simulink model "P702_NI_SoftECU"  (R2019a)
settings: Solver=ode1  StartTime=0.0  StopTime=Inf  FixedStep=0.001  RelTol=1e-3  EnableMultiTasking=on
PreLoadFcn:
  | run '.\VeriStand_BlockSet\NIVeriStandAddPaths.m'
undefined symbols (not defined in the file or in its folder): magnitude
libraries: simulink x83, simulink_extras x1
(part 42 of 76)

== system P702_NI_SoftECU/Input/Carsim/Bus Conversion/MRR_BUS1 ==
  In1 : Inport
  Bus Creator : BusCreator  Inputs=12
  Bus Selector : BusSelector  OutputSignals=CAN_DET_RANGE_01[m],CAN_DET_RANGE_RATE_01[m/s],CAN_DET_AZIMUTH_01[rad],CAN_DET_ELEVATION_01[rad],CAN_DET_RANGE_02[m],CAN_DET_RANGE_RATE_02[m/s],CAN_DET_AZIMUTH_02[rad],CAN_DET_ELEVATION_02[rad],CAN_DET_RANGE_03[m],CAN_DET_RANGE_RATE_03[m/s],CAN_DET_AZIMUTH_03[rad],CAN_DET_ELEVATION_03[rad]
  Gain : Gain  Commented=through  Gain=1/3.6
  Gain10 : Gain  Commented=through  Gain=pi/180
  Gain11 : Gain
  Gain12 : Gain  Commented=through  Gain=1/3.6
  Gain13 : Gain
  Gain14 : Gain  Commented=through  Gain=1/3.6
  Gain3 : Gain
  Gain6 : Gain  Commented=through  Gain=pi/180
  Gain9 : Gain  Commented=through  Gain=pi/180
  Out1 : Outport
  wires:
  Bus Selector/1 -> Bus Creator/1  "<CAN_DET_RANGE_01[m]>"
  Bus Selector/11 -> Gain11/1  "<CAN_DET_AZIMUTH_03[rad]>"
  Bus Selector/3 -> Gain3/1  "<CAN_DET_AZIMUTH_01[rad]>"
  Bus Selector/2 -> Gain/1  "<CAN_DET_RANGE_RATE_01[m/s]>"
  Bus Selector/7 -> Gain13/1  "<CAN_DET_AZIMUTH_02[rad]>"
  Bus Selector/6 -> Gain14/1  "<CAN_DET_RANGE_RATE_02[m/s]>"
  Bus Selector/9 -> Bus Creator/9  "<CAN_DET_RANGE_03[m]>"
  Bus Selector/5 -> Bus Creator/5  "<CAN_DET_RANGE_02[m]>"
  Bus Creator/1 -> Out1/1
  In1/1 -> Bus Selector/1
  Bus Selector/4 -> Gain10/1  "<CAN_DET_ELEVATION_01[rad]>"
  Bus Selector/12 -> Gain6/1  "<CAN_DET_ELEVATION_03[rad]>"
  Bus Selector/8 -> Gain9/1  "<CAN_DET_ELEVATION_02[rad]>"
  Gain/1 -> Bus Creator/2  "CAN_DET_RANGE_RATE_01[m/s]"
  Gain3/1 -> Bus Creator/3  "CAN_DET_AZIMUTH_01[rad]"
  Gain10/1 -> Bus Creator/4  "CAN_DET_ELEVATION_01[rad]"
  Gain14/1 -> Bus Creator/6  "CAN_DET_RANGE_RATE_02[m/s]"
  Gain13/1 -> Bus Creator/7  "CAN_DET_AZIMUTH_02[rad]"
  Gain9/1 -> Bus Creator/8  "CAN_DET_ELEVATION_02[rad]"
  Gain12/1 -> Bus Creator/10  "CAN_DET_RANGE_RATE_03[m/s]"
  Gain11/1 -> Bus Creator/11  "CAN_DET_AZIMUTH_03[rad]"
  Gain6/1 -> Bus Creator/12  "CAN_DET_ELEVATION_03[rad]"
  Bus Selector/10 -> Gain12/1  "<CAN_DET_RANGE_RATE_03[m/s]>"

== system P702_NI_SoftECU/Input/Carsim/Bus Conversion/PCM_BUS ==
  In1 : Inport
  BrkLightSwtch_B : Constant  Value=0
  Bus Creator : BusCreator  Inputs=8
  Bus Selector : BusSelector  OutputSignals=Throttle[percentage],V_total_Vehicle[km/h],Engine_RPM[rpm],Gear[],T_Engine[Nm],a_x_veh_COG[g]
  CluBottomOfTravelSwtch_B : Constant  Value=0
  Gain : Gain  Gain=100
  Gain1 : Gain  Gain=9.8
  Out1 : Outport
  wires:
  In1/1 -> Bus Selector/1
  Gain/1 -> Bus Creator/1  "Throttle[percentage]"
  BrkLightSwtch_B/1 -> Bus Creator/8  "BrkLightSwtch_B"
  CluBottomOfTravelSwtch_B/1 -> Bus Creator/7  "CluBottomOfTravelSwtch_B"
  Bus Creator/1 -> Out1/1
  Bus Selector/5 -> Bus Creator/5  "<T_Engine[Nm]>"
  Bus Selector/4 -> Bus Creator/4  "<Gear[]>"
  Bus Selector/3 -> Bus Creator/3  "<Engine_RPM[rpm]>"
  Bus Selector/2 -> Bus Creator/2  "<V_total_Vehicle[km/h]>"
  Bus Selector/1 -> Gain/1  "<Throttle[percentage]>"
  Bus Selector/6 -> Gain1/1  "<a_x_veh_COG[g]>"
  Gain1/1 -> Bus Creator/6  "a_x_veh_COG[m/s2]"

== system P702_NI_SoftECU/Input/Carsim/Bus Conversion/PCM_BUS1 ==
  In1 : Inport
  BrkLightSwtch_B : Constant  Value=0
  Bus Creator : BusCreator  Inputs=9
  Bus Selector : BusSelector  OutputSignals=Throttle[percentage],V_total_Vehicle[km/h],Engine_RPM[rpm],Gear[],T_Engine[Nm],a_x_veh_COG[g],MRR
  CluBottomOfTravelSwtch_B : Constant  Value=0
  Gain : Gain  Gain=100
  Gain1 : Gain
  Gain2 : Gain  Gain=3.6
  Gain3 : Gain  Gain=30/pi
  Out1 : Outport
  wires:
  In1/1 -> Bus Selector/1
  Gain/1 -> Bus Creator/1  "Throttle[percentage]"
  BrkLightSwtch_B/1 -> Bus Creator/8  "BrkLightSwtch_B"
  CluBottomOfTravelSwtch_B/1 -> Bus Creator/7  "CluBottomOfTravelSwtch_B"
  Bus Creator/1 -> Out1/1
  Bus Selector/5 -> Bus Creator/5  "<T_Engine[Nm]>"
  Bus Selector/4 -> Bus Creator/4  "<Gear[]>"
  Bus Selector/3 -> Gain3/1  "<Engine_RPM[rpm]>"
  Bus Selector/2 -> Gain2/1  "<V_total_Vehicle[km/h]>"
  Bus Selector/1 -> Gain/1  "<Throttle[percentage]>"
  Bus Selector/6 -> Gain1/1  "<a_x_veh_COG[g]>"
  Gain1/1 -> Bus Creator/6  "a_x_veh_COG[m/s2]"
  Gain2/1 -> Bus Creator/2  "V_total_Vehicle[km/h]"
  Gain3/1 -> Bus Creator/3  "Engine_RPM[rpm]"
  Bus Selector/7 -> Bus Creator/9  "<MRR>"

== system P702_NI_SoftECU/Input/Carsim/Bus Conversion/PSCM_BUS ==
  In1 : Inport
  Bus Creator : BusCreator  Inputs=1
  Bus Selector : BusSelector  OutputSignals=Agnle_SteeringWheel[deg]
  Out1 : Outport
  wires:
  Bus Creator/1 -> Out1/1
  Bus Selector/1 -> Bus Creator/1  "<Agnle_SteeringWheel[deg]>"
  In1/1 -> Bus Selector/1

== system P702_NI_SoftECU/Input/Carsim/Bus Conversion/PSCM_BUS1 ==
  In1 : Inport
  Bus Creator : BusCreator  Inputs=1
  Bus Selector : BusSelector  OutputSignals=Agnle_SteeringWheel[deg]
  Gain : Gain  Gain=180/pi
  Out1 : Outport
  wires:
  Bus Creator/1 -> Out1/1
  Bus Selector/1 -> Gain/1  "<Agnle_SteeringWheel[deg]>"
  In1/1 -> Bus Selector/1
  Gain/1 -> Bus Creator/1  "Agnle_SteeringWheel[deg]"

== system P702_NI_SoftECU/Input/Carsim/Bus Conversion/RCM_BUS ==
  In1 : Inport
  Bus Creator : BusCreator  Inputs=5
  Bus Selector : BusSelector  OutputSignals=RollRate_Veh_COG[deg/s],YawRate_Veh_COG[deg/s],a_x_veh_COG[g],a_y_veh_COG[g],a_z_Veh_COG[g]
  Gain1 : Gain  Gain=9.8
  Gain2 : Gain  Gain=9.8
  Gain3 : Gain  Gain=9.8
  Out1 : Outport
  wires:
  Bus Selector/1 -> Bus Creator/1  "<RollRate_Veh_COG[deg/s]>"
  Bus Selector/2 -> Bus Creator/2  "<YawRate_Veh_COG[deg/s]>"
  Bus Selector/5 -> Gain3/1  "<a_z_Veh_COG[g]>"
  Bus Selector/4 -> Gain2/1  "<a_y_veh_COG[g]>"
  Bus Selector/3 -> Gain1/1  "<a_x_veh_COG[g]>"
  Bus Creator/1 -> Out1/1
  In1/1 -> Bus Selector/1
  Gain1/1 -> Bus Creator/3  "a_x_veh_COG[m/s2]"
  Gain2/1 -> Bus Creator/4  "a_y_veh_COG[m/s2]"
  Gain3/1 -> Bus Creator/5  "a_z_Veh_COG[m/s2]"

== system P702_NI_SoftECU/Input/Carsim/Bus Conversion/RCM_BUS1 ==
  In1 : Inport
  Bus Creator : BusCreator  Inputs=5
  Bus Selector : BusSelector  OutputSignals=RollRate_Veh_COG[deg/s],YawRate_Veh_COG[deg/s],a_x_veh_COG[g],a_y_veh_COG[g],a_z_Veh_COG[g]
  Gain1 : Gain
  Gain2 : Gain
  Gain3 : Gain
  Gain4 : Gain  Gain=180/pi
  Gain5 : Gain  Gain=180/pi
  Out1 : Outport
  wires:
  Bus Selector/1 -> Gain4/1  "<RollRate_Veh_COG[deg/s]>"
  Bus Selector/2 -> Gain5/1  "<YawRate_Veh_COG[deg/s]>"
  Bus Selector/5 -> Gain3/1  "<a_z_Veh_COG[g]>"
  Bus Selector/4 -> Gain2/1  "<a_y_veh_COG[g]>"
  Bus Selector/3 -> Gain1/1  "<a_x_veh_COG[g]>"
  Bus Creator/1 -> Out1/1
  In1/1 -> Bus Selector/1
  Gain1/1 -> Bus Creator/3  "a_x_veh_COG[m/s2]"
  Gain2/1 -> Bus Creator/4  "a_y_veh_COG[m/s2]"
  Gain3/1 -> Bus Creator/5  "a_z_Veh_COG[m/s2]"
  Gain4/1 -> Bus Creator/1  "RollRate_Veh_COG[deg/s]"
  Gain5/1 -> Bus Creator/2  "YawRate_Veh_COG[deg/s]"

== system P702_NI_SoftECU/Input/Carsim/Bus Conversion/SCCM_BUS ==
  In1 : Inport
  Bus Creator : BusCreator  Inputs=4
  Bus Selector : BusSelector  OutputSignals=Pos_Z_veh[m],angle_Yaw[deg],Pos_veh_long[deg],Pos_veh_lat[deg]
  Out1 : Outport
  wires:
  Bus Creator/1 -> Out1/1
  Bus Selector/4 -> Bus Creator/4  "<Pos_veh_lat[deg]>"
  Bus Selector/3 -> Bus Creator/3  "<Pos_veh_long[deg]>"
  Bus Selector/2 -> Bus Creator/2  "<angle_Yaw[deg]>"
  Bus Selector/1 -> Bus Creator/1  "<Pos_Z_veh[m]>"
  In1/1 -> Bus Selector/1

== system P702_NI_SoftECU/Input/Carsim/Bus Conversion/SCCM_BUS1 ==
  In1 : Inport
  Bus Creator : BusCreator  Inputs=4
  Bus Selector : BusSelector  OutputSignals=Pos_Z_veh[m],angle_Yaw[deg],Pos_veh_long[deg],Pos_veh_lat[deg]
  Gain : Gain  Gain=180/pi
  Gain1 : Gain  Gain=180/pi
  Gain2 : Gain  Gain=180/pi
  Out1 : Outport
  wires:
  Bus Creator/1 -> Out1/1
  Bus Selector/4 -> Gain2/1  "<Pos_veh_lat[deg]>"
  Bus Selector/3 -> Gain1/1  "<Pos_veh_long[deg]>"
  Bus Selector/2 -> Gain/1  "<angle_Yaw[deg]>"
  Bus Selector/1 -> Bus Creator/1  "<Pos_Z_veh[m]>"
  In1/1 -> Bus Selector/1
  Gain/1 -> Bus Creator/2  "<angle_Yaw[deg]>"
  Gain1/1 -> Bus Creator/3  "<Pos_veh_long[deg]>"
  Gain2/1 -> Bus Creator/4  "<Pos_veh_lat[deg]>"

== system P702_NI_SoftECU/Input/Carsim/Bus Conversion/SRR_L_BUS ==
  In1 : Inport
  Bus Creator : BusCreator  Inputs=12
  Bus Selector : BusSelector  OutputSignals=SRR_L_DET_RANGE_01[m],SRR_L_DET_RANGE_RATE_01[m/s],SRR_L_DET_AZIMUTH_01[rad],SRR_L_DET_ELEVATION_01[rad],SRR_L_DET_RANGE_02[m],SRR_L_DET_RANGE_RATE_02[m/s],SRR_L_DET_AZIMUTH_02[rad],SRR_L_DET_ELEVATION_02[rad],SRR_L_DET_RANGE_03[m],SRR_L_DET_RANGE_RATE_03[m/s],SRR_L_DET_AZIMUTH_03[rad],SRR_L_DET_ELEVATION_03[rad]
  Gain : Gain  Commented=through  Gain=1/3.6
  Gain10 : Gain  Commented=through  Gain=pi/180
  Gain11 : Gain
  Gain12 : Gain  Commented=through  Gain=1/3.6
  Gain13 : Gain
  Gain14 : Gain  Commented=through  Gain=1/3.6
  Gain3 : Gain
  Gain6 : Gain  Commented=through  Gain=pi/180
  Gain9 : Gain  Commented=through  Gain=pi/180
  Out1 : Outport
  wires:
  Bus Selector/1 -> Bus Creator/1  "<SRR_L_DET_RANGE_01[m]>"
  Bus Selector/11 -> Gain11/1  "<SRR_L_DET_AZIMUTH_03[rad]>"
  Bus Selector/3 -> Gain3/1  "<SRR_L_DET_AZIMUTH_01[rad]>"
  Bus Selector/2 -> Gain/1  "<SRR_L_DET_RANGE_RATE_01[m/s]>"
  Bus Selector/7 -> Gain13/1  "<SRR_L_DET_AZIMUTH_02[rad]>"
  Bus Selector/6 -> Gain14/1  "<SRR_L_DET_RANGE_RATE_02[m/s]>"
  Bus Selector/9 -> Bus Creator/9  "<SRR_L_DET_RANGE_03[m]>"
  Bus Selector/5 -> Bus Creator/5  "<SRR_L_DET_RANGE_02[m]>"
  Bus Creator/1 -> Out1/1
  In1/1 -> Bus Selector/1
  Bus Selector/4 -> Gain10/1  "<SRR_L_DET_ELEVATION_01[rad]>"
  Bus Selector/12 -> Gain6/1  "<SRR_L_DET_ELEVATION_03[rad]>"
  Bus Selector/8 -> Gain9/1  "<SRR_L_DET_ELEVATION_02[rad]>"
  Gain/1 -> Bus Creator/2  "SRR_L_DET_RANGE_RATE_01[m/s]"
  Gain3/1 -> Bus Creator/3  "SRR_L_DET_AZIMUTH_01[rad]"
  Gain10/1 -> Bus Creator/4  "SRR_L_DET_ELEVATION_01[rad]"
  Gain14/1 -> Bus Creator/6  "SRR_L_DET_RANGE_RATE_02[m/s]"
  Gain13/1 -> Bus Creator/7  "SRR_L_DET_AZIMUTH_02[rad]"
  Gain9/1 -> Bus Creator/8  "SRR_L_DET_ELEVATION_02[rad]"
  Gain12/1 -> Bus Creator/10  "SRR_L_DET_RANGE_RATE_03[m/s]"
  Gain11/1 -> Bus Creator/11  "SRR_L_DET_AZIMUTH_03[rad]"
  Gain6/1 -> Bus Creator/12  "SRR_L_DET_ELEVATION_03[rad]"
  Bus Selector/10 -> Gain12/1  "<SRR_L_DET_RANGE_RATE_03[m/s]>"

== system P702_NI_SoftECU/Input/Carsim/Bus Conversion/SRR_R_BUS ==
  In1 : Inport
  Bus Creator : BusCreator  Inputs=12
  Bus Selector : BusSelector  OutputSignals=SRR_R_DET_RANGE_01[m],SRR_R_DET_RANGE_RATE_01[m/s],SRR_R_DET_AZIMUTH_01[rad],SRR_R_DET_ELEVATION_01[rad],SRR_R_DET_RANGE_02[m],SRR_R_DET_RANGE_RATE_02[m/s],SRR_R_DET_AZIMUTH_02[rad],SRR_R_DET_ELEVATION_02[rad],SRR_R_DET_RANGE_03[m],SRR_R_DET_RANGE_RATE_03[m/s],SRR_R_DET_AZIMUTH_03[rad],SRR_R_DET_ELEVATION_03[rad]
  Gain : Gain  Commented=through  Gain=1/3.6
  Gain10 : Gain  Commented=through  Gain=pi/180
  Gain11 : Gain
  Gain12 : Gain  Commented=through  Gain=1/3.6
  Gain13 : Gain
  Gain14 : Gain  Commented=through  Gain=1/3.6
  Gain3 : Gain
  Gain6 : Gain  Commented=through  Gain=pi/180
  Gain9 : Gain  Commented=through  Gain=pi/180
  Out1 : Outport
  wires:
  Bus Selector/10 -> Gain12/1  "<SRR_R_DET_RANGE_RATE_03[m/s]>"
  Gain6/1 -> Bus Creator/12  "SRR_R_DET_ELEVATION_03[rad]"
  Gain11/1 -> Bus Creator/11  "SRR_R_DET_AZIMUTH_03[rad]"
  Gain12/1 -> Bus Creator/10  "SRR_R_DET_RANGE_RATE_03[m/s]"
  Gain9/1 -> Bus Creator/8  "SRR_R_DET_ELEVATION_02[rad]"
  Gain13/1 -> Bus Creator/7  "SRR_R_DET_AZIMUTH_02[rad]"
  Gain14/1 -> Bus Creator/6  "SRR_R_DET_RANGE_RATE_02[m/s]"
  Gain10/1 -> Bus Creator/4  "SRR_R_DET_ELEVATION_01[rad]"
  Gain3/1 -> Bus Creator/3  "SRR_R_DET_AZIMUTH_01[rad]"
  Bus Selector/8 -> Gain9/1  "<SRR_R_DET_ELEVATION_02[rad]>"
  Bus Selector/12 -> Gain6/1  "<SRR_R_DET_ELEVATION_03[rad]>"
  Bus Selector/4 -> Gain10/1  "<SRR_R_DET_ELEVATION_01[rad]>"
  In1/1 -> Bus Selector/1
  Bus Creator/1 -> Out1/1
  Bus Selector/5 -> Bus Creator/5  "<SRR_R_DET_RANGE_02[m]>"
  Bus Selector/9 -> Bus Creator/9  "<SRR_R_DET_RANGE_03[m]>"
  Bus Selector/6 -> Gain14/1  "<SRR_R_DET_RANGE_RATE_02[m/s]>"
  Bus Selector/7 -> Gain13/1  "<SRR_R_DET_AZIMUTH_02[rad]>"
  Bus Selector/2 -> Gain/1  "<SRR_R_DET_RANGE_RATE_01[m/s]>"
  Bus Selector/3 -> Gain3/1  "<SRR_R_DET_AZIMUTH_01[rad]>"
  Bus Selector/11 -> Gain11/1  "<SRR_R_DET_AZIMUTH_03[rad]>"
  Bus Selector/1 -> Bus Creator/1  "<SRR_R_DET_RANGE_01[m]>"
  Gain/1 -> Bus Creator/2  "SRR_R_DET_RANGE_RATE_01[m/s]"

== system P702_NI_SoftECU/Input/Carsim/Bus Conversion/TCM_BUS ==
  In1 : Inport
  Bus Creator : BusCreator  Inputs=1
  Bus Selector : BusSelector  OutputSignals=Gear_Lever_POS[]
  Out1 : Outport
  tag scope: Gear_Lvr_Position=global
  wires:
  Bus Creator/1 -> Out1/1
  Bus Selector/1 -> Bus Creator/1, [Gear_Lvr_Position]  "<Gear_Lever_POS[]>"
  In1/1 -> Bus Selector/1

== system P702_NI_SoftECU/Input/Carsim/Bus Conversion/TCM_BUS1 ==
  In1 : Inport
  Bus Creator : BusCreator  Inputs=1
  Bus Selector : BusSelector  OutputSignals=Gear_Lever_POS[]
  Out1 : Outport
  tag scope: Gear_Lvr_Position=global
  wires:
  Bus Creator/1 -> Out1/1
  Bus Selector/1 -> Bus Creator/1, [Gear_Lvr_Position]  "<Gear_Lever_POS[]>"
  In1/1 -> Bus Selector/1

== system P702_NI_SoftECU/Input/GWM-SCCM//PDB//RCM//GSM/GSM/Gear_Shift_by_Wire_2_FD1 ==
  Bus_Sig : BusCreator  Inputs=4
  GearButtnStuck_B_Actl : S-Function  Priority=1  FunctionName=NIVeriStandIO  Parameters=width dtype portnum stime stype btype  SFunctionDeploymentMode=off  EnableBusSupport=off  mask(NI VeriStand Inport){portnum=1, width=-1, stime=-1, dtype=auto, stype=auto, btype=1}
      mask prompts: portnum "Port number:"; width "Port dimensions (-1 for dynamically sized):"; stime "Sample time (-1 for inherited):"; dtype "Data type:"; stype "Signal type:"; btype "Block type:"
      mask help: Use this inport on any level of nested subsystems to allow NI VeriStand software to map signals to it.
      mask init:
      | NIVeriStandIO_init;
      settings: CopyFcn=NIVeriStand_MDL_functions('', 'IO_copy');  DeleteFcn=NIVeriStand_MDL_functions('', 'IO_delete');  MoveFcn=set_param(gcb, 'Mask', 'on');
      mask Callback portnum: NIVeriStand_MDL_functions('', 'IO_setportnum');
      mask TypeOptions dtype: auto | double | single | int8 | uint8 | int16 | uint16 | int32 | uint32 | boolean
      mask Callback dtype: NIVeriStand_MDL_functions('', 'IO_booleansignal');
      mask TypeOptions stype: auto | real | complex
      mask Display:
      | patch([-x x], [-y y], [.90980 .81960 .32156]);
      | plot([xrad -x x xrad], [yrad -y y yrad]);
      | fprintf('NI In%d', portnum);
  GsmSrvcRqd_B_Rq : S-Function  Priority=2  FunctionName=NIVeriStandIO  Parameters=width dtype portnum stime stype btype  SFunctionDeploymentMode=off  EnableBusSupport=off  mask(NI VeriStand Inport){portnum=2, width=-1, stime=-1, dtype=auto, stype=auto, btype=1}
      mask prompts: portnum "Port number:"; width "Port dimensions (-1 for dynamically sized):"; stime "Sample time (-1 for inherited):"; dtype "Data type:"; stype "Signal type:"; btype "Block type:"
      mask help: Use this inport on any level of nested subsystems to allow NI VeriStand software to map signals to it.
      mask init:
      | NIVeriStandIO_init;
      settings: CopyFcn=NIVeriStand_MDL_functions('', 'IO_copy');  DeleteFcn=NIVeriStand_MDL_functions('', 'IO_delete');  MoveFcn=set_param(gcb, 'Mask', 'on');
      mask Callback portnum: NIVeriStand_MDL_functions('', 'IO_setportnum');
      mask TypeOptions dtype: auto | double | single | int8 | uint8 | int16 | uint16 | int32 | uint32 | boolean
      mask Callback dtype: NIVeriStand_MDL_functions('', 'IO_booleansignal');
      mask TypeOptions stype: auto | real | complex
      mask Display:
      | patch([-x x], [-y y], [.90980 .81960 .32156]);
      | plot([xrad -x x xrad], [yrad -y y yrad]);
      | fprintf('NI In%d', portnum);
  TrnGearPwmFalt_B_Actl : S-Function  Priority=3  FunctionName=NIVeriStandIO  Parameters=width dtype portnum stime stype btype  SFunctionDeploymentMode=off  EnableBusSupport=off  mask(NI VeriStand Inport){portnum=3, width=-1, stime=-1, dtype=auto, stype=auto, btype=1}
      mask prompts: portnum "Port number:"; width "Port dimensions (-1 for dynamically sized):"; stime "Sample time (-1 for inherited):"; dtype "Data type:"; stype "Signal type:"; btype "Block type:"
      mask help: Use this inport on any level of nested subsystems to allow NI VeriStand software to map signals to it.
      mask init:
      | NIVeriStandIO_init;
      settings: CopyFcn=NIVeriStand_MDL_functions('', 'IO_copy');  DeleteFcn=NIVeriStand_MDL_functions('', 'IO_delete');  MoveFcn=set_param(gcb, 'Mask', 'on');
      mask Callback portnum: NIVeriStand_MDL_functions('', 'IO_setportnum');
      mask TypeOptions dtype: auto | double | single | int8 | uint8 | int16 | uint16 | int32 | uint32 | boolean
      mask Callback dtype: NIVeriStand_MDL_functions('', 'IO_booleansignal');
      mask TypeOptions stype: auto | real | complex
      mask Display:
      | patch([-x x], [-y y], [.90980 .81960 .32156]);
      | plot([xrad -x x xrad], [yrad -y y yrad]);
      | fprintf('NI In%d', portnum);
  TrnTrcmPwmSig_D_Actl : S-Function  Priority=4  FunctionName=NIVeriStandIO  Parameters=width dtype portnum stime stype btype  SFunctionDeploymentMode=off  EnableBusSupport=off  mask(NI VeriStand Inport){portnum=4, width=-1, stime=-1, dtype=auto, stype=auto, btype=1}
      mask prompts: portnum "Port number:"; width "Port dimensions (-1 for dynamically sized):"; stime "Sample time (-1 for inherited):"; dtype "Data type:"; stype "Signal type:"; btype "Block type:"
      mask help: Use this inport on any level of nested subsystems to allow NI VeriStand software to map signals to it.
      mask init:
      | NIVeriStandIO_init;
      settings: CopyFcn=NIVeriStand_MDL_functions('', 'IO_copy');  DeleteFcn=NIVeriStand_MDL_functions('', 'IO_delete');  MoveFcn=set_param(gcb, 'Mask', 'on');
      mask Callback portnum: NIVeriStand_MDL_functions('', 'IO_setportnum');
      mask TypeOptions dtype: auto | double | single | int8 | uint8 | int16 | uint16 | int32 | uint32 | boolean
      mask Callback dtype: NIVeriStand_MDL_functions('', 'IO_booleansignal');
      mask TypeOptions stype: auto | real | complex
      mask Display:
      | patch([-x x], [-y y], [.90980 .81960 .32156]);
      | plot([xrad -x x xrad], [yrad -y y yrad]);
      | fprintf('NI In%d', portnum);
  Gear_Shift_by_Wire_2_FD1_168 : Outport
  wires:
  Bus_Sig/1 -> Gear_Shift_by_Wire_2_FD1_168/1  "Gear_Shift_by_Wire_2_FD1_168"
  GearButtnStuck_B_Actl/1 -> Bus_Sig/1  "GearButtnStuck_B_Actl"
  GsmSrvcRqd_B_Rq/1 -> Bus_Sig/2  "GsmSrvcRqd_B_Rq"
  TrnGearPwmFalt_B_Actl/1 -> Bus_Sig/3  "TrnGearPwmFalt_B_Actl"
  TrnTrcmPwmSig_D_Actl/1 -> Bus_Sig/4  "TrnTrcmPwmSig_D_Actl"
